simulink model "quadcopter_package_delivery"  (R2024a)
settings: Solver=ode23t  StartTime=0.0  StopTime=timespot_spl(end)+4  FixedStep=0.01  MaxStep=1e-2  RelTol=1e-3  AbsTol=1e-3
PostLoadFcn:
  | warning('off','sm:sli:setup:compile:LocalSolverNotSupported')
undefined symbols (not defined in the file): A, B, battery_capacity, filtD_motor, filtD_position, filtM_position, filtSpd_motor, kd_motor, kd_position, ki_motor, ki_position, kp_motor, kp_position, limit_motor, pkgDensity, planedepth, pos2attitude, qd_area, qd_drag, spline_data, spline_yaw, timespot_spl, waypoints, X, Y, Z
libraries: sm_lib x67, nesl_utility x35, fl_lib x13, slpidlib x8, quadcopter_library x6, ee_lib x4, slctrl_adaptive x1, batteryecm_lib x1
(part 4 of 4)

== system quadcopter_package_delivery/Quadcopter/Body/Aerodynamic Drag/drag force Y ==
  Constant : Constant  Value=rho_air/2
  Constant1 : Constant  Value=area_values.XZ
  Constant2 : Constant  Value=drag_coeff.Cd_Y
  Gain : Gain  Gain=-1
  PS-Simulink Converter : nesl_utility/PS-Simulink Converter  PhysicalDomain=network_engine_domain  SubClassName=ps_output  LeftPortType=input  RightPortType=output  PseudoPeriodic=off  Frequencies=[]  VectorFormat=1-D array  Unit=inherit  AffineConversion=off
  Product : Product  Inputs=5
  Sign : Signum  ZeroCross=off
  Simulink-PS Converter : nesl_utility/Simulink-PS Converter  PhysicalDomain=network_engine_domain  SubClassName=ps_input  LeftPortType=input  RightPortType=output  PseudoPeriodic=off  Frequencies=[]  NoiseDistribution=none  NoiseParameters=[]  Unit=1  AffineConversion=off  FilteringAndDerivatives=provide  SimscapeFilterOrder=1  InputFilterTimeConstant=0.001  UdotUserProvided=0
  Square : Math  Operator=square
  vel : PMIOPort  Side=Right
  fdrag : PMIOPort  Port=2  Side=Left
  wires:
  PS-Simulink Converter/1 -> Sign/1, Square/1
  Constant1/1 -> Product/2
  Sign/1 -> Product/5
  Gain/1 -> Simulink-PS Converter/1
  Constant2/1 -> Product/3
  Square/1 -> Product/4
  Product/1 -> Gain/1
  Constant/1 -> Product/1
  connections:
  Simulink-PS Converter/RConn1 -- fdrag/RConn1
  vel/RConn1 -- PS-Simulink Converter/LConn1

== system quadcopter_package_delivery/Quadcopter/Body/Aerodynamic Drag/drag force Z ==
  Constant : Constant  Value=rho_air/2
  Constant1 : Constant  Value=area_values.XY
  Constant2 : Constant  Value=drag_coeff.Cd_Z
  Gain : Gain  Gain=-1
  PS-Simulink Converter : nesl_utility/PS-Simulink Converter  PhysicalDomain=network_engine_domain  SubClassName=ps_output  LeftPortType=input  RightPortType=output  PseudoPeriodic=off  Frequencies=[]  VectorFormat=1-D array  Unit=inherit  AffineConversion=off
  Product : Product  Inputs=5
  Sign : Signum  ZeroCross=off
  Simulink-PS Converter : nesl_utility/Simulink-PS Converter  PhysicalDomain=network_engine_domain  SubClassName=ps_input  LeftPortType=input  RightPortType=output  PseudoPeriodic=off  Frequencies=[]  NoiseDistribution=none  NoiseParameters=[]  Unit=1  AffineConversion=off  FilteringAndDerivatives=provide  SimscapeFilterOrder=1  InputFilterTimeConstant=0.001  UdotUserProvided=0
  Square : Math  Operator=square
  vel : PMIOPort  Side=Right
  fdrag : PMIOPort  Port=2  Side=Left
  wires:
  PS-Simulink Converter/1 -> Sign/1, Square/1
  Gain/1 -> Simulink-PS Converter/1
  Square/1 -> Product/4
  Product/1 -> Gain/1
  Sign/1 -> Product/5
  Constant1/1 -> Product/2
  Constant/1 -> Product/1
  Constant2/1 -> Product/3
  connections:
  Simulink-PS Converter/RConn1 -- fdrag/RConn1
  vel/RConn1 -- PS-Simulink Converter/LConn1

== system quadcopter_package_delivery/Quadcopter/Body/Aerodynamic Drag/drag moment pitch ==
  Constant : Constant  Value=rho_air/2
  Constant1 : Constant  Value=area_values.Pitch
  Constant2 : Constant  Value=drag_coeff.Pitch
  Gain : Gain  Gain=-1
  PS-Simulink Converter : nesl_utility/PS-Simulink Converter  PhysicalDomain=network_engine_domain  SubClassName=ps_output  LeftPortType=input  RightPortType=output  PseudoPeriodic=off  Frequencies=[]  VectorFormat=1-D array  Unit=inherit  AffineConversion=off
  Product : Product  Inputs=5
  Sign : Signum  ZeroCross=off
  Simulink-PS Converter : nesl_utility/Simulink-PS Converter  PhysicalDomain=network_engine_domain  SubClassName=ps_input  LeftPortType=input  RightPortType=output  PseudoPeriodic=off  Frequencies=[]  NoiseDistribution=none  NoiseParameters=[]  Unit=1  AffineConversion=off  FilteringAndDerivatives=provide  SimscapeFilterOrder=1  InputFilterTimeConstant=0.001  UdotUserProvided=0
  Square : Math  Operator=square
  vel : PMIOPort  Side=Right
  fdrag : PMIOPort  Port=2  Side=Left
  wires:
  Product/1 -> Gain/1
  Constant2/1 -> Product/3
  PS-Simulink Converter/1 -> Sign/1, Square/1
  Constant/1 -> Product/1
  Sign/1 -> Product/5
  Constant1/1 -> Product/2
  Gain/1 -> Simulink-PS Converter/1
  Square/1 -> Product/4
  connections:
  Simulink-PS Converter/RConn1 -- fdrag/RConn1
  vel/RConn1 -- PS-Simulink Converter/LConn1

== system quadcopter_package_delivery/Quadcopter/Body/Aerodynamic Drag/drag moment roll ==
  Constant : Constant  Value=rho_air/2
  Constant1 : Constant  Value=area_values.Roll
  Constant2 : Constant  Value=drag_coeff.Roll
  Gain : Gain  Gain=-1
  PS-Simulink Converter : nesl_utility/PS-Simulink Converter  PhysicalDomain=network_engine_domain  SubClassName=ps_output  LeftPortType=input  RightPortType=output  PseudoPeriodic=off  Frequencies=[]  VectorFormat=1-D array  Unit=inherit  AffineConversion=off
  Product : Product  Inputs=5
  Sign : Signum  ZeroCross=off
  Simulink-PS Converter : nesl_utility/Simulink-PS Converter  PhysicalDomain=network_engine_domain  SubClassName=ps_input  LeftPortType=input  RightPortType=output  PseudoPeriodic=off  Frequencies=[]  NoiseDistribution=none  NoiseParameters=[]  Unit=1  AffineConversion=off  FilteringAndDerivatives=provide  SimscapeFilterOrder=1  InputFilterTimeConstant=0.001  UdotUserProvided=0
  Square : Math  Operator=square
  vel : PMIOPort  Side=Right
  fdrag : PMIOPort  Port=2  Side=Left
  wires:
  Product/1 -> Gain/1
  PS-Simulink Converter/1 -> Sign/1, Square/1
  Constant/1 -> Product/1
  Constant1/1 -> Product/2
  Constant2/1 -> Product/3
  Square/1 -> Product/4
  Sign/1 -> Product/5
  Gain/1 -> Simulink-PS Converter/1
  connections:
  Simulink-PS Converter/RConn1 -- fdrag/RConn1
  PS-Simulink Converter/LConn1 -- vel/RConn1

== system quadcopter_package_delivery/Quadcopter/Body/Aerodynamic Drag/drag moment yaw ==
  Constant : Constant  Value=rho_air/2
  Constant1 : Constant  Value=area_values.Yaw
  Constant2 : Constant  Value=drag_coeff.Yaw
  Gain : Gain  Gain=-1
  PS-Simulink Converter : nesl_utility/PS-Simulink Converter  PhysicalDomain=network_engine_domain  SubClassName=ps_output  LeftPortType=input  RightPortType=output  PseudoPeriodic=off  Frequencies=[]  VectorFormat=1-D array  Unit=inherit  AffineConversion=off
  Product : Product  Inputs=5
  Sign : Signum  ZeroCross=off
  Simulink-PS Converter : nesl_utility/Simulink-PS Converter  PhysicalDomain=network_engine_domain  SubClassName=ps_input  LeftPortType=input  RightPortType=output  PseudoPeriodic=off  Frequencies=[]  NoiseDistribution=none  NoiseParameters=[]  Unit=1  AffineConversion=off  FilteringAndDerivatives=provide  SimscapeFilterOrder=1  InputFilterTimeConstant=0.001  UdotUserProvided=0
  Square : Math  Operator=square
  vel : PMIOPort  Side=Right
  fdrag : PMIOPort  Port=2  Side=Left
  wires:
  Constant1/1 -> Product/2
  Sign/1 -> Product/5
  Constant/1 -> Product/1
  PS-Simulink Converter/1 -> Sign/1, Square/1
  Gain/1 -> Simulink-PS Converter/1
  Constant2/1 -> Product/3
  Square/1 -> Product/4
  Product/1 -> Gain/1
  connections:
  Simulink-PS Converter/RConn1 -- fdrag/RConn1
  vel/RConn1 -- PS-Simulink Converter/LConn1

== matlab function quadcopter_package_delivery/Maneuver Controller/Outer-Loop-Position Control/Calculate RBI ==
  data: R_BI output; attitude input
function R_BI  = Calculate_RBI(attitude)

phi   = attitude(1);
theta = attitude(2);
psi   = attitude(3);

% obtain the desired state
R_BI = [cos(theta)*cos(psi)                                    cos(theta)*sin(psi)                          -sin(theta);
    -cos(phi)*sin(psi)+sin(phi)*sin(theta)*cos(psi) cos(phi)*cos(psi)+sin(phi)*sin(theta)*sin(psi) sin(phi)*cos(theta);
    sin(phi)*sin(psi)+cos(phi)*sin(theta)*cos(psi) -sin(phi)*cos(psi)+cos(phi)*sin(theta)*sin(psi) cos(phi)*cos(theta)];

end
